simulink model "ex_400"  (R2018b)
settings: Solver=VariableStepAuto  StartTime=0.0  StopTime=2  FixedStep=0.0001  RelTol=1e-3
settings Model: Creator=lenovo  LastModifiedBy=QJ-
settings DebuggingCC: LibraryContextMissingDiagnostic=none
settings SFSimCC: SimUseLocalCustomCode=off
settings RTWCC: RTWUseLocalCustomCode=off

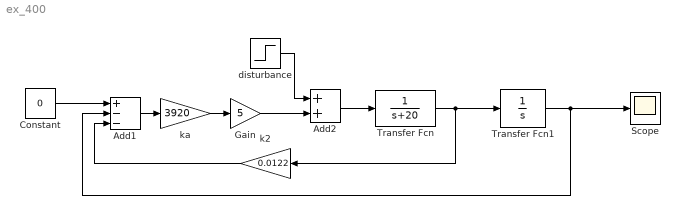
== system ex_400 ==
  Add1 : Sum  Inputs=+--
  Add2 : Sum
  Constant : Constant  Value=0
  Gain : Gain  Gain=5
  Scope : Scope
  Transfer Fcn : TransferFcn  Denominator=[1 20]
  Transfer Fcn1 : TransferFcn  Denominator=[1 0]
  disturbance : Step  Time=0  SampleTime=1  mask(DiscretizedSource){}
      mask init:
      | %zoh
  k2 : Gain  Gain=0.0122
  ka : Gain  Gain=3920
  wires:
  Transfer Fcn1/1 -> Scope/1, Add1/2
  Add1/1 -> ka/1
  k2/1 -> Add1/3
  ka/1 -> Gain/1
  Transfer Fcn/1 -> k2/1, Transfer Fcn1/1
  Gain/1 -> Add2/2
  Add2/1 -> Transfer Fcn/1
  disturbance/1 -> Add2/1
  Constant/1 -> Add1/1
